simulink model "delayToRam"  (R2024a)
settings: Solver=FixedStepDiscrete  StartTime=0.0  StopTime=2000/100e6  RelTol=1e-3
settings Model: DataTypeOverride=Off  Creator=cotti  LastModifiedBy=cotti
settings OptimizationCC: BlockReduction=off  ConditionallyExecuteInputs=off  DefaultParameterBehavior=Inlined  InheritOutputTypeSmallerThanSingle=on
settings DebuggingCC: AlgebraicLoopMsg=error  ArtificialAlgebraicLoopMsg=error  SingleTaskRateTransMsg=error  UnconnectedInputMsg=warning  UnconnectedOutputMsg=warning  UnconnectedLineMsg=warning
settings HardwareCC: ProdBitPerPointer=32  ProdBitPerSizeT=32  ProdBitPerPtrDiffT=32  ProdLargestAtomicFloat=None  ProdIntDivRoundTo=Undefined  ProdEndianess=Unspecified  ProdWordSize=32  ProdHWDeviceType=ASIC/FPGA->ASIC/FPGA  TargetBitPerLong=64  TargetBitPerPointer=64  TargetBitPerSizeT=64  TargetBitPerPtrDiffT=64  TargetLongLongMode=on  TargetIntDivRoundTo=Zero  TargetEndianess=LittleEndian  TargetWordSize=64  TargetHWDeviceType=Custom Processor->MATLAB Host Computer  ProdEqTarget=off

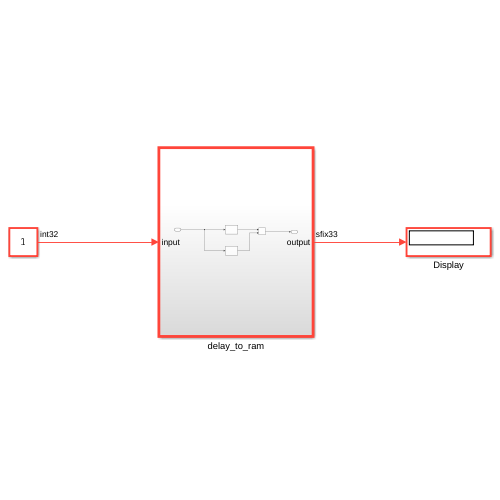
[thumbnail: Simulink's stored preview of the top-level diagram]
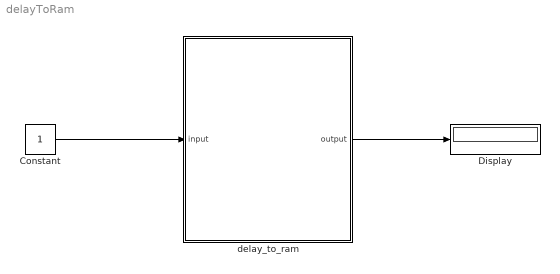
== system delayToRam ==
  Constant : Constant  OutDataTypeStr=int32  SampleTime=1/100e6
  Display : Display
  delay_to_ram : Subsystem  TreatAsAtomicUnit=on
  wires:
  Constant/1 -> delay_to_ram/1(input)
  delay_to_ram/1(output) -> Display/1

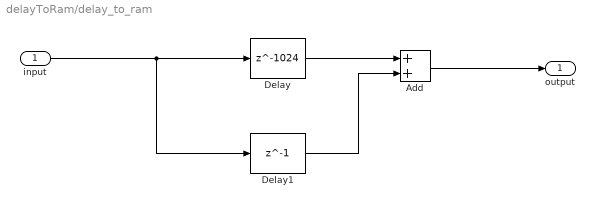
== system delayToRam/delay_to_ram ==
  input : Inport
  Add : Sum
  Delay : Delay  DelayLength=1024  InitialCondition=0  UseCircularBuffer=on
  Delay1 : Delay  DelayLength=1  InitialCondition=0  UseCircularBuffer=on
  output : Outport
  wires:
  input/1 -> Delay1/1, Delay/1
  Delay/1 -> Add/1
  Delay1/1 -> Add/2
  Add/1 -> output/1
